simulink subsystem "BAM_Controller"  (R2026a)
settings: Solver=VariableStepAuto
undefined symbols (not defined in the file): DiscIntNeverNeededParam, SimIn, SimPar
libraries: simulink x11, starslibMathOperations x2, sharedTrackingLibrary x1, simulink_extras x1, starslibAxisTransformations x1
(part 3 of 3)

== matlab function BAM_Controller/Avoidance Planner/Ball is Moving/Trajectory Planning ==
  data: t_now input; DesTraj input Bus: BUS_USER_Traj_Iner; flagMode input; clearFlag input; dbRelTraj input; d_traj input; safeTraj output Bus: BUS_USER_Traj_Iner; mode output; D_cmd output; n_avoid_dbg output; missDistNorm input; bb_traj input
function [safeTraj, ...
          mode, ...
          D_cmd, ...
          n_avoid_dbg] ...
    = safeTraj( ...
          t_now, ...
          DesTraj, ...
          flagMode, ...
          clearFlag, ...
          dbRelTraj, ...
          d_traj, ...
		  missDistNorm, ...
          bb_traj)

% THE FOLLOWING PREAMBLE IS AI
%{
BLOCK DIAGRAM / LOGIC OVERVIEW
------------------------------
This planner is a finite-state machine that generates a lateral avoidance
offset for the drone to avoid an incoming ball while preserving a smooth
trajectory.

INPUTS
------
flagMode   : threat/avoidance trigger
             0 = no active avoidance request
             1 = avoidance requested

clearFlag  : return-to-nominal trigger
             0 = keep avoiding
             1 = obstacle/threat is considered clear

D_des      : desired avoidance distance based on current ball geometry
n_hat      : nominal lateral direction
n_ball     : ball-relative direction used to choose avoidance side
t          : current time

INTERNAL MEMORY (persistent)
----------------------------
state      : current planner mode
t_state    : time when current state started
D0         : avoidance offset at start of transition
D_target   : target avoidance offset for current maneuver
n_avoid    : latched avoidance direction
T_state    : transition duration

STATE DEFINITIONS
-----------------
state = 0  -> NOMINAL
             Drone follows nominal path with no avoidance offset.

state = 1  -> BLEND OUT
             Drone smoothly transitions from nominal path to avoidance
             offset using quintic blending.

state = 2  -> HOLD OFFSET
             Drone holds the commanded avoidance offset.

state = 3  -> BLEND BACK
             Drone smoothly returns from avoidance offset to nominal path.

HIGH-LEVEL FLOW
---------------
                +-------------------+
                |   Inputs:         |
                | flagMode          |
                | clearFlag         |
                | D_des, n_hat      |
                | n_ball, t         |
                +---------+---------+
                          |
                          v
                +-------------------+
                |  Choose/update    |
                |  avoidance side   |
                |  and target       |
                +---------+---------+
                          |
                          v
                +-------------------+
                |  State Machine    |
                |  switch(state)    |
                +---------+---------+
                          |
      +-------------------+-------------------+
      |                   |                   |
      v                   v                   v
+-----------+      +-------------+     +-------------+
| state 0   | ---> | state 1     | --> | state 2     |
| NOMINAL   |      | BLEND OUT   |     | HOLD OFFSET |
+-----------+      +-------------+     +-------------+
      ^                   |                   |
      |                   v                   v
      |             +-------------+ <---------+
      +-------------| state 3     |
                    | BLEND BACK  |
                    +-------------+

STATE TRANSITIONS
-----------------
0 -> 1 : flagMode == 1
         Start avoidance. Latch avoidance direction n_avoid, set D_target,
         store transition start time.

1 -> 2 : blend-out complete
         Avoidance offset has reached target; hold it.

1 -> 3 : clearFlag == 1
         Threat cleared before full offset is reached; begin return.

2 -> 1 : flagMode == 1 and D_des > D_target
         Threat persists or worsens; increase avoidance offset and blend again.

2 -> 3 : clearFlag == 1
         Threat cleared; begin return to nominal path.

3 -> 0 : blend-back complete
         Return to nominal flight.

3 -> 1 : flagMode == 1
         New threat appears while returning; re-enter avoidance.

OUTPUT BEHAVIOR
---------------
The planner outputs a smooth lateral avoidance command:
    nominal path
      + blended avoidance offset in direction n_avoid

The offset magnitude is:
    0 in state 0,
    increasing in state 1,
    held near D_target in state 2,
    decreasing back to 0 in state 3.

DESIGN INTENT
-------------
- Prevent abrupt path jumps by using time-based blending.
- Hold avoidance while the threat remains active.
- Return smoothly to nominal once clear.
- Re-enter avoidance immediately if a new threat appears.
%}
% END OF AI :)


% Pull apart

pos_i = DesTraj.pos_i;
vel_i = DesTraj.vel_i;
acc_i = DesTraj.acc_i;

pos_bi = d_traj(1:3, :);
vel_bi = d_traj(1:3, :);

relBPos = dbRelTraj(1:3, 1);
ballVel = bb_traj(4:6, :);

% Define Initials

R_safe = 3;
buffer = 0.75;
D_min = 1;
D_max = 4;
T_out = .6;
T_back = .6;

resetPlanner = 0;

% Make Persistent

persistent ...
	state ...
	n_avoid ...
	t_state ...
	D_start ...
	D_target ...
	T_state
	
% States:
%   0 = nominal
%   1 = blend out
%   2 = hold offset
%   3 = blend back

% Initialize
if isempty(state)
	state = int32(0);
	n_avoid = [0; 0; 0];
	t_state = 0;
	D_start = 0;
	D_target = 0;
	T_state = 0;
end
	
if resetPlanner
	state = int32(0);
	n_avoid = [0; 0; 0];
	t_state = t_now;
	D_start = 0;
	D_target = 0;
	T_state = 1;
end

% switch to column vectors for consistency
pos_i = pos_i(:);
vel_i = vel_i(:);
acc_i = acc_i(:);
pos_bi = pos_bi(:);
vel_bi = vel_bi(:);
relBPos = relBPos(:);
ballVel = ballVel(:);

% Defaults
pos_cmd = pos_i;
vel_cmd = vel_i;
acc_cmd = acc_i;
mode = state;
D_cmd = 0;
eps_norm = 1e-6;

% ----- Compute avoidance Direction ----- %
% Prefer perpendicular to current drone heading, away from ball

v_body = vel_bi;
v_ball = ballVel;

if norm(v_body) > eps_norm
	e_v = v_body / norm(v_body);
elseif norm(vel_i) > eps_norm
    e_v = vel_i / norm(vel_i);
else
    e_v = [1; 0; 0];
end

v_rel = v_ball - v_body; % Relative motion

% dont move along current heading
n_candidate = v_rel - dot(v_rel, e_v) * e_v;
if norm(n_candidate) < eps_norm
    n_candidate = relBPos - dot(relBPos, e_v) * e_v;
end

% pick new, nonaligned axis for heading
if norm(n_candidate) < eps_norm
    if abs(e_v(3)) < 0.9
        axis_ref = [0; 0; 1];
    else
        axis_ref = [0; 1; 0];
    end
    n_candidate = axis_ref - dot(axis_ref, e_v) * e_v;
end

n_candidate = n_candidate / max(norm(n_candidate), eps_norm);

% move away from ball by flipping the sign if needed
if dot(n_candidate, relBPos) > 0
    n_candidate = -n_candidate;
end

% ----- Offset Magnitude ----- %
% adds margin to normal miss distance
D_des = max(D_min, (R_safe + buffer - missDistNorm));
D_des = min(D_des, D_max);

% ----- Quintic Calculations for D_dot/D_ddot ----- %
% We compute current D, D_dot, D_ddot from the stored transition.
D_now    = 0.0;
D_dot    = 0.0;
D_ddot   = 0.0;

if state == 1 || state == 3
    T_use = max(T_state, 1e-3);
    s = (t_now - t_state) / T_use;

    % Quintic blend with explicit 3 cases:
    % case A: s <= 0
    % case B: 0 < s < 1
    % case C: s >= 1
    if s <= 0
        alpha    = 0.0;
        alpha_d  = 0.0;
        alpha_dd = 0.0;
    elseif s < 1
        alpha    = 10*s^3 - 15*s^4 + 6*s^5;
        alpha_d  = 30*s^2 - 60*s^3 + 30*s^4;
        alpha_dd = 60*s   - 180*s^2 + 120*s^3;
    else
        alpha    = 1.0;
        alpha_d  = 0.0;
        alpha_dd = 0.0;
    end

    dDelta = D_target - D_start;

    D_now  = D_start + dDelta * alpha;
    D_dot  = dDelta * alpha_d  / T_use;
    D_ddot = dDelta * alpha_dd / (T_use^2);
elseif state == 2
    D_now  = D_target;
    D_dot  = 0.0;
    D_ddot = 0.0;
else
    D_now  = 0.0;
    D_dot  = 0.0;
    D_ddot = 0.0;
end

% ----- Different switch cases ----- %
% Need to have cases to go in and out of different states in case  
% the sensors miss something, that way were not locked into one path

switch state
	case 0 
		% nominal
		D_now = 0;
		D_dot = 0;
		D_ddot = 0;
		
		if flagMode
			% latch avoidance once
			n_avoid = n_candidate;
			
			% transition out
			D_start = 0;
			D_target = D_des;
			T_state = max(T_out, 1e-3);
			t_state = t_now;
			state = int32(1);
		end
	
	case 1 
		% Blend out
		
		if clearFlag
			% Go back to blend back
			D_start = D_now;
			D_target = 0;
			T_state = max(T_back, 1e-3);
			t_state = t_now;
			state = int32(3);
		else
			% expand offset if threat is still bad
			if D_des > D_target
				D_start = D_now;
				D_target = D_des;
				T_state = max(.5 * T_out, 1e-3);
				t_state = t_now;
				state = int32(1);
			end
			
			if (t_now - t_state) >= T_state
				% blend out time is done, hold offset
				D_now = D_target;
				D_dot = 0;
				D_ddot = 0;
				D_start = D_target;
				state = int32(2);
			end
		end
		
	case 2 
		% Hold offset
		D_now = D_target;
		D_dot = 0;
		D_ddot = 0;
		
		if clearFlag
			% Return to nominal
			D_start = D_now;
			D_target = 0;
			T_state = max(T_back, 1e-3);
			t_state = t_now;
			state = int32(3);
		else
			% expand offset if threat is still bad
			if flagMode && (D_des > D_target)
				D_start = D_now;
				D_target = D_des;
				T_state = max(.5 * T_out, 1e-3);
				t_state = t_now;
				state = int32(1);
			end
		end
		
	case 3
		% Blend back
		if flagMode && ~clearFlag
			% Blend out again
			n_avoid = n_candidate;
			D_start = D_now;
			D_target = max(D_now, D_des);
			T_state = max(T_out, 1e-3);
			t_state = t_now;
			state = int32(1);
		else
			% back to nominal
			if (t_now - t_state) >= T_state
				D_now = 0;
				D_dot = 0;
				D_ddot = 0;
				D_start = 0;
				D_target = 0;
				state = int32(0);
			end
		end
	
	otherwise
		n_avoid = [0; 0; 0];
		t_state = t_now;
		T_state = 1;
		D_now = 0;
		D_dot = 0;
		D_ddot = 0;
		D_start = 0;
		D_target = 0;
		state = int32(0);
end

% -----	Calculate commands, produce outputs ----- %
pos_cmd = pos_i + n_avoid * D_now;
vel_cmd = vel_i + n_avoid * D_dot;
acc_cmd = acc_i + n_avoid * D_ddot;

safeTraj = DesTraj;

% New safeTraj
safeTraj.pos_i = pos_cmd;
safeTraj.vel_i = vel_cmd;
safeTraj.acc_i = acc_cmd;

% Debug outputs
mode = state;
D_cmd = D_now;
n_avoid_dbg = n_avoid;

== matlab function BAM_Controller/Avoidance Planner/Ball is Moving/Set Covariances ==
  data: bb_traj input; R_out output; Q_out output
function [R_out, Q_out] = setCov(bb_traj)
persistent Rf Qf liveTime init

dt = 1/200;

R_out = zeros(3,3);
Q_out = zeros(6,6);

% Velocity and position breakdown
px = bb_traj(1,1);
py = bb_traj(2,1);
pz = bb_traj(3,1);
vx = bb_traj(4,1);
vy = bb_traj(5,1);
vz = bb_traj(6,1);

% Initialize Setup at start
if isempty(init)
    q0 = diag([.01, .01, .01, .1, .1, .1]);
    r0 = diag([1, 1, 1]);

    Qf = q0;
    Rf = r0;
    liveTime = 0;
    init = true;
end

T_warmup = 0.01;
beta = 0.98; % For low pass
qv_min = 1e-4; % Keep EKF from using 0
r_min = 1e-4;

% Calculate Sensor Noise (Q)
Q_noise = 0.1; % how much of the noise to constrain to
v_mag_now = sqrt(vx ^2 + vy ^2 + vz ^2);
v_noise = max(Q_noise * v_mag_now, qv_min);

Q_calc = diag([0.1, 0.1, 0.1, v_noise, v_noise, v_noise]);

% Calculate Measurement Noise (R)

R_noise = 0.1; % Based on the NOISER
Px_sdsq = max((R_noise * px)^2, r_min);
Py_sdsq = max((R_noise * py)^2, r_min);
Pz_sdsq = max((R_noise * pz)^2, r_min);

R_calc = diag([Px_sdsq, Py_sdsq, Pz_sdsq]);

% Warmup logic
if liveTime * dt <= T_warmup
    % hold startup values
else
    Qf = beta * Qf + (1 - beta) * Q_calc;
    Rf = beta * Rf + (1 - beta) * R_calc;
end

% Output w/ symmetry, increase liveTime
Q_out = 0.5 * (Qf + Qf.');
R_out = 0.5 * (Rf + Rf.');

% disp(Q_out)
% disp(R_out)

liveTime = liveTime + 1;

end

== matlab function BAM_Controller/Path-following control/Body-Inertial Rotation Matrix/MATLAB Function ==
  data: q input; R output
function R = qToRot(q)

q0 = q(1); q1 = q(2); q2 = q(3); q3 = q(4);

R11 = q0^2 + q1^2 - q2^2 - q3^2;
R12 = 2*( q1*q2 + q0*q3 );
R13 = 2*( q1*q3 - q0*q2 );

R21 = 2*( q1*q2 - q0*q3 );
R22 = q0^2 - q1^2 + q2^2 - q3^2;
R23 = 2*( q2*q3 + q0*q1 );

R31 = 2*( q1*q3 + q0*q2 );
R32 = 2*( q2*q3 - q0*q1 );
R33 = q0^2 - q1^2 - q2^2 + q3^2;

R = [R11 R12 R13; R21 R22 R23; R31 R32 R33];

== matlab function BAM_Controller/Avoidance Planner/Ball is Moving/MATLAB Function1 ==
  data: bb_traj input; px output; py output; pz output; vx output; vy output; vz output
function [px,py, pz, vx, vy, vz] = fcn(bb_traj)

px = bb_traj(1,1);
py = bb_traj(2,1);
pz = bb_traj(3,1);
vx = bb_traj(4,1);
vy = bb_traj(5,1);
vz = bb_traj(6,1);

end

== matlab function BAM_Controller/Path-following control/Desired Frame/MATLAB Function ==
  data: R input; rpy output
function rpy = RotToEuler(R)

p = -asin(R(1,3));
r = atan2(R(2,3),R(3,3));
y = atan2(R(1,2),R(1,1));

rpy = [r p y]';

== matlab function BAM_Controller/Path-following control/Path/Heading Hold Logic prevents badness when trajectory is vertical/Heading Vector in Horz Plane/MATLAB Function ==
  data: q input; R output
function R = qToRot(q)

q0 = q(1); q1 = q(2); q2 = q(3); q3 = q(4);

R11 = q0^2 + q1^2 - q2^2 - q3^2;
R12 = 2*( q1*q2 + q0*q3 );
R13 = 2*( q1*q3 - q0*q2 );

R21 = 2*( q1*q2 - q0*q3 );
R22 = q0^2 - q1^2 + q2^2 - q3^2;
R23 = 2*( q2*q3 + q0*q1 );

R31 = 2*( q1*q3 + q0*q2 );
R32 = 2*( q2*q3 - q0*q1 );
R33 = q0^2 - q1^2 - q2^2 + q3^2;

R = [R11 R12 R13; R21 R22 R23; R31 R32 R33];

== matlab function BAM_Controller/Path-following control/Path/Heading Hold Logic prevents badness when trajectory is vertical/Heading Vector in Horz Plane/MATLAB Function1 ==
  data: quat_input input; euler_output output
% Jan Vervoorst, vervoors@illinois.edu
% University of Illinois 2015/16
%--------------------------------------------------------------------------
%% Find  roll, pitch, yaw from quaternion
% This files takes a quaternion as input and transforms it 
% into Roll/Pitch/Yaw Euler angles.
% Representative of Euler angle sequence (1,2,3) according to
% "Representing Attitude: Euler Angles, Unit Quaternions, and Rotation Vectors"
% by James Diebel, Stanford University, 20 October 2006
%--------------------------------------------------------------------------
function euler_output = quat2rpy(quat_input)
%-------------------------------------------------------
% System states
q0 = quat_input(1); % Quaternion input 0
q1 = quat_input(2); % Quaternion input 1
q2 = quat_input(3); % Quaternion input 2
q3 = quat_input(4); % Quaternion input 3
%-------------------------------------------------------
% This is the (1,2,3) angle sequence computation:
roll  = atan2(2*q2*q3+2*q0*q1,q3^2-q2^2-q1^2+q0^2);
pitch = -asin(2*q1*q3-2*q0*q2);
yaw   = atan2(2*q1*q2+2*q0*q3,q1^2+q0^2-q3^2-q2^2); 
%-------------------------------------------------------
% Outputs are the three Euler angles Roll, Pitch, Yaw
euler_output = zeros(3,1);
euler_output(1) = roll;
euler_output(2) = pitch;
euler_output(3) = yaw;
%--------------------------------------------------------------------------
% end of file

== matlab function BAM_Controller/Path-following control/omega_c/MATLAB Function1 ==
  data: M input; v output
function v = vee_map(M)
%#codegen

% if any([M(1,1), M(2,2), M(3,3), M(1,2)+M(2,1), M(1,3)+M(3,1), M(2,3)+M(3,2)])
%     warning('M is not an element of SO(3). Results may not be valid.')
% end

v = [0; 0; 0;];

v(1) = M(3,2);
v(2) = M(1,3);
v(3) = M(2,1);

== matlab function BAM_Controller/Path-following control/omega_c/MATLAB Function3 ==
  data: M input; v output
function v = vee_map(M)
%#codegen

% if any([M(1,1), M(2,2), M(3,3), M(1,2)+M(2,1), M(1,3)+M(3,1), M(2,3)+M(3,2)])
%     warning('M is not an element of SO(3). Results may not be valid.')
% end

v = [0; 0; 0;];

v(1) = M(3,2);
v(2) = M(1,3);
v(3) = M(2,1);

== matlab function BAM_Controller/Path-following control/Path/Heading Hold Logic prevents badness when trajectory is vertical/Heading Vector in Horz Plane/MATLAB Function4 ==
  data: quat_input input; quat_output output
% Jan Vervoorst, vervoors@illinois.edu
% University of Illinois 2015/16
%--------------------------------------------------------------------------
%% Find quaternion from roll, pitch, yaw
%  This files takes Roll/Pitch/Yaw Euler angles as inputs
% and transforms into the quaternion representation.
% Representative of Euler angle sequence (1,2,3) according to
% "Representing Attitude: Euler Angles, Unit Quaternions, and Rotation Vectors"
% by James Diebel, Stanford University, 20 October 2006
%--------------------------------------------------------------------------
function quat_output = rpy2quat(quat_input)
%-------------------------------------------------------
% System states
roll  = quat_input(1);  % Roll input [rad]
pitch = quat_input(2);  % Pitch input [rad]
yaw   = quat_input(3);  % Yaw input [rad]
%-------------------------------------------------------
phi   = roll / 2;
theta = pitch / 2;
psi   = yaw / 2;
%
cphi   = cos(phi);
sphi   = sin(phi);
ctheta = cos(theta);
stheta = sin(theta);
cpsi   = cos(psi);
spsi   = sin(psi);
%
% This is the (1,2,3) angle sequence computation:
q0 = cphi * ctheta * cpsi + sphi * stheta * spsi;
q1 = sphi * ctheta * cpsi - cphi * stheta * spsi;
q2 = cphi * stheta * cpsi + sphi * ctheta * spsi;
q3 = cphi * ctheta * spsi - sphi * stheta * cpsi;
%-------------------------------------------------------	
if (q0 < 0.0)       % q0 always positive for uniqueness of the quaternion
    q0 = -q0;
	q1 = -q1;
	q2 = -q2;
	q3 = -q3;
end
%-------------------------------------------------------
% Outputs are the four entries of the desired normalized attitude quaternion
quat_output = zeros(4,1);
quat_output(1,1) = q0;
quat_output(2,1) = q1;
quat_output(3,1) = q2;
quat_output(4,1) = q3;
%--------------------------------------------------------------------------
% end of file
